simulink model "minseg_balanced"  (R2024a)
settings: Solver=FixedStepAuto  StartTime=0.0  StopTime=inf  FixedStep=.003  RelTol=1e-3  EnableMultiTasking=on
values from neighbouring files (symbols this model uses):
  KLQR = lqr(A, B, Q, R)    [sim_minseg.m]
  Rw = 0.0216    [minseg.m]    (also in sim_minseg.m)
undefined symbols (not defined in the file or in its folder): DiscIntNeverNeededParam
libraries: arduinolib x4, simulink x3, arduinosensorlib x2
settings Model: ExtModeTrigDuration=2  Creator=hurstj  LastModifiedBy=Meenakshi Mahagaokar
settings DataIOCC: SaveOutput=off  DSMLogging=off  SaveTime=off  ReturnWorkspaceOutputs=off
settings OptimizationCC: EnhancedBackFolding=on  PassReuseOutputArgsThreshold=0  MaxStackSize=64  OptimizeBlockOrder=speed  DifferentSizesBufferReuse=on  OptimizationCustomize=off
settings DebuggingCC: ParameterTunabilityLossMsg=error
settings HardwareCC: ProdBitPerInt=16  ProdBitPerPointer=16  ProdBitPerSizeT=16  ProdBitPerPtrDiffT=16  ProdLargestAtomicFloat=None  ProdWordSize=8  ProdHWDeviceType=Atmel->AVR  UseEmbeddedCoderFeatures=off  UseSimulinkCoderFeatures=off
settings SFSimCC: MATLABDynamicMemAlloc=off
settings RTWCC: Description=Embedded Coder  SystemTargetFile=ert.tlc  HardwareBoard=Arduino Mega 2560  TemplateMakefile=ert_default_tmf  Toolchain=Arduino AVR  BuildConfiguration=Faster Runs  GPUComputeCapability=3.5
settings CodeAppCC: ForceParamTrailComments=on  OperatorAnnotations=on  MangleLength=10
settings ERTTargetCC: ERTCustomFileBanners=off  SupportContinuousTime=on  SupportNonInlinedSFcns=on  RemoveResetFunc=off  SupportVariableSizeSignals=on  ModelStepFunctionPrototypeControlCompliant=off  ExtModeTransport=3  ExtModeStaticAlloc=on  ExtModeAutomaticAllocSize=off  ExtModeStaticAllocSize=2048  ExtModeMexFile=ext_xcp  ExtModeIntrfLevel=Level2 - Open

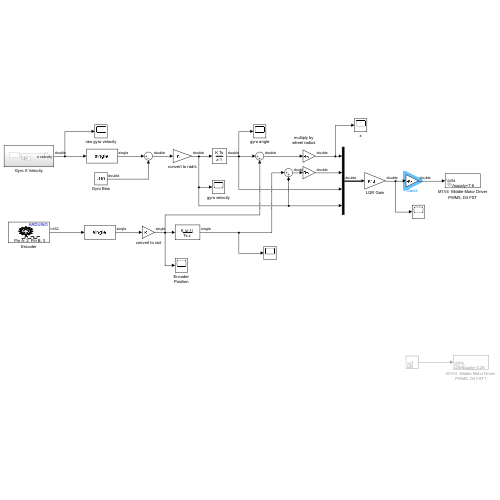
[thumbnail: Simulink's stored preview of the top-level diagram]
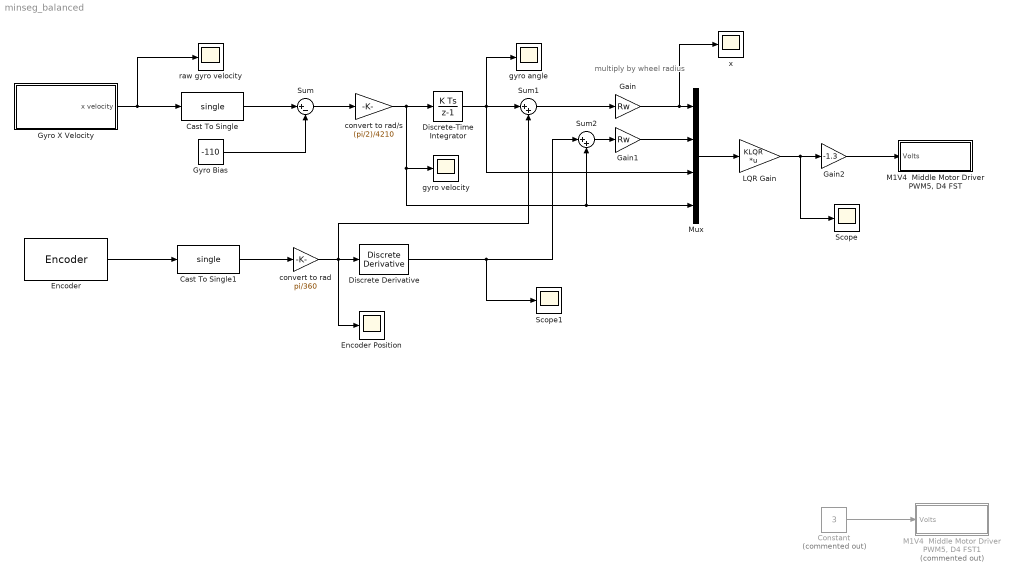
== system minseg_balanced ==
  note: multiply by
      | wheel radius
  Cast To Single : DataTypeConversion  OutDataTypeStr=single  SaturateOnIntegerOverflow=off  RndMeth=Floor
  Cast To Single1 : DataTypeConversion  OutDataTypeStr=single  SaturateOnIntegerOverflow=off  RndMeth=Floor
  Constant : Constant  Commented=on  Value=3
  Discrete Derivative : simulink/Discrete/Discrete Derivative  gainval=1.0  ICPrevScaledInput=0.0  OutMin=[]  OutMax=[]  OutDataType=fixdt(1, 16)  OutScaling=2^-10  DoSatur=off
  Discrete-Time Integrator : DiscreteIntegrator  SampleTime=-1  ICPrevOutput=DiscIntNeverNeededParam  ICPrevScaledInput=DiscIntNeverNeededParam
  Encoder : arduinosensorlib/Encoder  InputA=2  InputB=3  Mode=No reset  SampleTime=.003
  Encoder Position : Scope
  Gain : Gain  Gain=Rw
  Gain1 : Gain  Gain=Rw
  Gain2 : Gain  Gain=-1.3
  Gyro Bias : Constant  Value=-110
  Gyro X Velocity : Subsystem
  LQR Gain : Gain  Gain=KLQR  Multiplication=Matrix(K*u)
  "M1V4  Middle Motor Driver PWM5, D4 FST" : Subsystem  mask(Motor Driver){Vsupply=7.6}
      mask prompts: Vsupply "Driver Supply Voltage"
      mask help:
      | Use a single PWM and a single Digtial out to control the magnitude and direction of a motor
      |
      | Specify driver supply voltage (~3.25 for USB with SN754410)
      |
      | Driver supply voltage can be measured direcly by turning the motor fully on (100% duty cycle) and measuring the voltage across the motor leads.  This is the maximum voltage available to the motor and is used to scale from volts to PWM value 0-255.
      |
      | Note this value must be changed if the supply voltage to the driver is changed, for example, by using batteries.
      |
      | Vsupply is the maximum voltage your system is capable of supplying to system given the power supply. It needs to be measured depending on the power supply.
      mask Display:
      | port_label('input',1,'Volts')
      | text(15,5,['Vsupply=' num2str(Vsupply)])
  "M1V4  Middle Motor Driver PWM5, D4 FST1" : Subsystem  Commented=on  mask(Motor Driver){Vsupply=3.25}
      mask prompts: Vsupply "Driver Supply Voltage"
      mask help:
      | Use a single PWM and a single Digtial out to control the magnitude and direction of a motor
      |
      | Specify driver supply voltage (~3.25 for USB with SN754410)
      |
      | Driver supply voltage can be measured direcly by turning the motor fully on (100% duty cycle) and measuring the voltage across the motor leads.  This is the maximum voltage available to the motor and is used to scale from volts to PWM value 0-255.
      |
      | Note this value must be changed if the supply voltage to the driver is changed, for example, by using batteries.
      |
      | Vsupply is the maximum voltage your system is capable of supplying to system given the power supply. It needs to be measured depending on the power supply.
      mask Display:
      | port_label('input',1,'Volts')
      | text(15,5,['Vsupply=' num2str(Vsupply)])
  Mux : Mux
  Scope : Scope
  Scope1 : Scope
  Sum : Sum  Inputs=|+-
  Sum1 : Sum  Inputs=|++
  Sum2 : Sum  Inputs=|++
  convert to rad : Gain  Gain=pi/360
  convert to rad/s : Gain  Gain=(pi/2)/4210
  gyro angle : Scope
  gyro velocity : Scope
  raw gyro velocity : Scope
  x : Scope
  wires:
  Gyro X Velocity/1(x velocity) -> raw gyro velocity/1, Cast To Single/1
  Cast To Single/1 -> Sum/1
  Gyro Bias/1 -> Sum/2
  Sum/1 -> convert to rad/s/1
  convert to rad/s/1 -> gyro velocity/1, Mux/4, Sum2/2, Discrete-Time Integrator/1
  Encoder/1 -> Cast To Single1/1
  Cast To Single1/1 -> convert to rad/1
  convert to rad/1 -> Discrete Derivative/1, Sum1/2, Encoder Position/1
  Mux/1 -> LQR Gain/1
  Discrete-Time Integrator/1 -> gyro angle/1, Mux/3, Sum1/1
  Gain/1 -> x/1, Mux/1
  Sum1/1 -> Gain/1
  Sum2/1 -> Gain1/1
  Gain1/1 -> Mux/2
  Discrete Derivative/1 -> Scope1/1, Sum2/1
  LQR Gain/1 -> Scope/1, Gain2/1
  Gain2/1 -> "M1V4  Middle Motor Driver PWM5, D4 FST"/1(Volts)
  Constant/1 -> "M1V4  Middle Motor Driver PWM5, D4 FST1"/1(Volts)

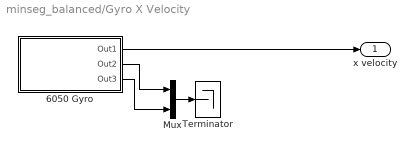
== system minseg_balanced/Gyro X Velocity ==
  6050 Gyro : Subsystem
      mask Display: disp('soMPU6050Gyro')
  Mux : Mux  Inputs=2
  Terminator : Terminator
  x velocity : Outport
  wires:
  6050 Gyro/2(Out2) -> Mux/1
  Mux/1 -> Terminator/1
  6050 Gyro/3(Out3) -> Mux/2
  6050 Gyro/1(Out1) -> x velocity/1

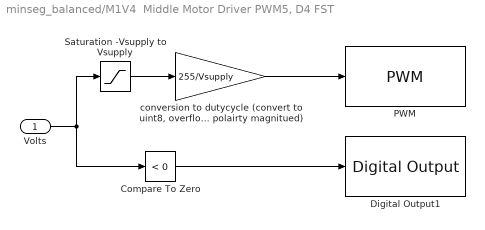
== system minseg_balanced/M1V4  Middle Motor Driver PWM5, D4 FST ==
  Volts : Inport
  Compare To Zero : simulink/Logic and Bit Operations/Compare To Zero  relop=<  OutDataTypeStr=boolean
  Digital Output1 : arduinolib/Digital Output  pinNumber=4  Direction=output  blockPlatform=arduino
  PWM : arduinolib/PWM  pinNumber=5  frequencyType=Default  desiredFrequency=490.2  achievableFrequency=490.2
  Saturation -Vsupply to Vsupply : Saturate  UpperLimit=Vsupply  LowerLimit=-Vsupply  OutDataTypeStr=single
  "conversion to dutycycle (convert to uint8, overflow will provide reverse polairty magnitued)" : Gain  Gain=255/Vsupply  OutDataTypeStr=uint8
  wires:
  Compare To Zero/1 -> Digital Output1/1
  "conversion to dutycycle (convert to uint8, overflow will provide reverse polairty magnitued)"/1 -> PWM/1
  Saturation -Vsupply to Vsupply/1 -> "conversion to dutycycle (convert to uint8, overflow will provide reverse polairty magnitued)"/1
  Volts/1 -> Saturation -Vsupply to Vsupply/1, Compare To Zero/1

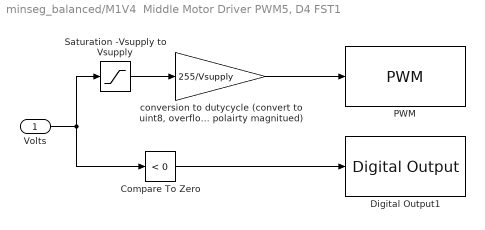
== system minseg_balanced/M1V4  Middle Motor Driver PWM5, D4 FST1 ==
  Volts : Inport
  Compare To Zero : simulink/Logic and Bit Operations/Compare To Zero  relop=<  OutDataTypeStr=boolean
  Digital Output1 : arduinolib/Digital Output  pinNumber=4  Direction=output  blockPlatform=arduino
  PWM : arduinolib/PWM  pinNumber=5  frequencyType=Default  desiredFrequency=490.2  achievableFrequency=490.2
  Saturation -Vsupply to Vsupply : Saturate  UpperLimit=Vsupply  LowerLimit=-Vsupply  OutDataTypeStr=single
  "conversion to dutycycle (convert to uint8, overflow will provide reverse polairty magnitued)" : Gain  Gain=255/Vsupply  OutDataTypeStr=uint8
  wires:
  Compare To Zero/1 -> Digital Output1/1
  "conversion to dutycycle (convert to uint8, overflow will provide reverse polairty magnitued)"/1 -> PWM/1
  Saturation -Vsupply to Vsupply/1 -> "conversion to dutycycle (convert to uint8, overflow will provide reverse polairty magnitued)"/1
  Volts/1 -> Saturation -Vsupply to Vsupply/1, Compare To Zero/1

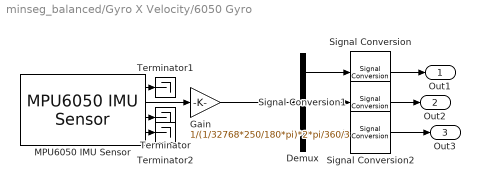
== system minseg_balanced/Gyro X Velocity/6050 Gyro ==
  Demux : Demux  Outputs=3
  Gain : Gain  Gain=1/(1/32768*250/180*pi)*2*pi/360/3
  MPU6050 IMU Sensor : arduinosensorlib/MPU6050 IMU Sensor  I2CModule=0  SlaveAddress=0x68  Accel=on  AngularRate=on  Temperature=on  Status=on  Timestamp=off  EulerAngles=off  Quat=off  AccelRange=2G  GyroRange=250 dps  DmpOdr=200 Hz  Dlpf=Accelerometer: 184Hz, Gyroscope: 188Hz  spf=1  SampleTime=-1  QueueSizeFactor=1
  Signal Conversion : SignalConversion  OverrideOpt=off
  Signal Conversion1 : SignalConversion  OverrideOpt=off
  Signal Conversion2 : SignalConversion  OverrideOpt=off
  Terminator : Terminator
  Terminator1 : Terminator
  Terminator2 : Terminator
  Out1 : Outport
  Out2 : Outport  Port=2
  Out3 : Outport  Port=3
  wires:
  Signal Conversion/1 -> Out1/1
  Signal Conversion2/1 -> Out3/1
  Signal Conversion1/1 -> Out2/1
  MPU6050 IMU Sensor/1 -> Terminator1/1
  Demux/2 -> Signal Conversion1/1
  Demux/3 -> Signal Conversion2/1
  Demux/1 -> Signal Conversion/1
  MPU6050 IMU Sensor/2 -> Gain/1
  MPU6050 IMU Sensor/4 -> Terminator2/1
  MPU6050 IMU Sensor/3 -> Terminator/1
  Gain/1 -> Demux/1
